simulink model "torqueBalancingSOT_logData"  (Simulink 8.8)
settings: Solver=FixedStepDiscrete  StartTime=0.0  StopTime=CONFIG.SIMULATION_TIME  FixedStep=CONFIG.Ts  RelTol=1e-3  EnableMultiTasking=on
InitFcn:
  | cd(fileparts(which(bdroot)));
  | initTorqueBalancingSOT;
undefined symbols (not defined in the file or in its folder): CONFIG, ConstraintsFeetMatrix, DiscIntNeverNeededParam, gain, reg, ROBOT_DOF, sat, sm, upperBoundFeetConstraints, WBT_robotName
libraries: WBToolboxLibrary x69
(part 2 of 2)

== system torqueBalancingSOT_logData/Visualize and log/Visualize torques ==
  state : Inport
  measuredJointsTorque : Inport  Port=2
  desiredJointsTorque : Inport  Port=3
  Enable : EnablePort
  Add : Sum  Inputs=+-
  DoFs converter : WBToolboxLibrary/Utilities/DoFs converter  yarp2WBIOption=From WBI to YARP  robotName=WBT_robotName  localName=WBT_modelName  wbiFile=WBT_wbiFilename  wbiList=WBT_wbiList
  DoFs converter1 : WBToolboxLibrary/Utilities/DoFs converter  yarp2WBIOption=From WBI to YARP  robotName=WBT_robotName  localName=WBT_modelName  wbiFile=WBT_wbiFilename  wbiList=WBT_wbiList
  DoFs converter2 : WBToolboxLibrary/Utilities/DoFs converter  yarp2WBIOption=From WBI to YARP  robotName=WBT_robotName  localName=WBT_modelName  wbiFile=WBT_wbiFilename  wbiList=WBT_wbiList
  desiredJointTorques : Scope  NumInputPorts=6
  errorJointTorques : Scope  NumInputPorts=6
  measuredJointTorques : Scope  NumInputPorts=6
  wires:
  DoFs converter1/2 -> desiredJointTorques/2  "left_arm"
  DoFs converter2/3 -> errorJointTorques/3  "right_arm"
  DoFs converter2/5 -> errorJointTorques/5  "right_leg"
  DoFs converter2/1 -> errorJointTorques/1  "torso"
  DoFs converter/5 -> measuredJointTorques/5  "right_leg"
  DoFs converter/4 -> measuredJointTorques/4  "left_leg"
  DoFs converter/2 -> measuredJointTorques/2  "left_arm"
  DoFs converter/1 -> measuredJointTorques/1  "torso"
  desiredJointsTorque/1 -> DoFs converter1/1, Add/2
  measuredJointsTorque/1 -> Add/1, DoFs converter/1
  DoFs converter/3 -> measuredJointTorques/3  "right_arm"
  DoFs converter2/4 -> errorJointTorques/4  "left_leg"
  DoFs converter1/1 -> desiredJointTorques/1  "torso"
  DoFs converter1/3 -> desiredJointTorques/3  "right_arm"
  DoFs converter1/4 -> desiredJointTorques/4  "left_leg"
  DoFs converter2/2 -> errorJointTorques/2  "left_arm"
  Add/1 -> DoFs converter2/1
  DoFs converter1/5 -> desiredJointTorques/5  "right_leg"
  state/1 -> measuredJointTorques/6, errorJointTorques/6, desiredJointTorques/6

== system torqueBalancingSOT_logData/synchronizer/GAZEBO_SYNCHRONIZER ==
  Enable : EnablePort
  Simulator Synchronizer : WBToolboxLibrary/Utilities/Simulator Synchronizer  period=CONFIG.Ts  serverPortName='/clock/rpc'  clientPortName='/WBT_synchronizer/rpc:o'

== system torqueBalancingSOT_logData/synchronizer/REAL_TIME_SYNC ==
  Enable : EnablePort
  Real Time Synchronizer : WBToolboxLibrary/Utilities/Real Time Synchronizer  period=CONFIG.Ts

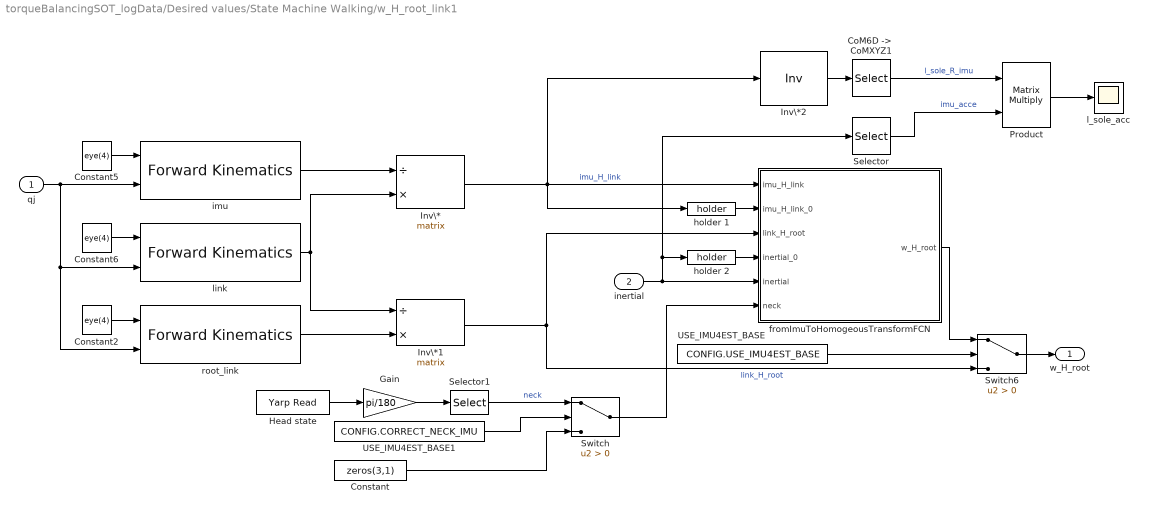
== system torqueBalancingSOT_logData/Desired values/State Machine Walking/w_H_root_link1 ==
  qj : Inport
  inertial : Inport  Port=2
  "CoM6D ->  CoMXYZ1" : Selector  NumberOfDimensions=2  InputPortWidth=7  IndexOptions=Index vector (dialog),Index vector (dialog)  Indices=[1 2 3],[1 2 3]  OutputSizes=1,1
  Constant : Constant  Value=zeros(3,1)
  Constant2 : Constant  Value=eye(4)
  Constant5 : Constant  Value=eye(4)
  Constant6 : Constant  Value=eye(4)
  Gain : Gain  Gain=pi/180
  Head state : WBToolboxLibrary/Utilities/Yarp Read  portName=[WBT_robotName, '/head/state:o']  signalSize=6  blocking=off  timestamp=off  autoconnect=on  errorOnConnection=off
  Inv\* : Product  Inputs=/*  Multiplication=Matrix(*)
  Inv\*1 : Product  Inputs=/*  Multiplication=Matrix(*)
  Inv\*2 : Product  Inputs=/  Multiplication=Matrix(*)
  Product : Product  Multiplication=Matrix(*)
  Selector : Selector  InputPortWidth=12  IndexOptions=Index vector (dialog)  Indices=[4 5 6 ]  OutputSizes=1
  Selector1 : Selector  InputPortWidth=6  IndexOptions=Index vector (dialog)  Indices=[1:3]  OutputSizes=1
  Switch : Switch  Criteria=u2 > Threshold
  Switch6 : Switch  Criteria=u2 > Threshold
  USE_IMU4EST_BASE : Constant  Value=CONFIG.USE_IMU4EST_BASE
  USE_IMU4EST_BASE1 : Constant  Value=CONFIG.CORRECT_NECK_IMU
  fromImuToHomogeousTransformFCN : MATLAB Function  TreatAsAtomicUnit=on
  holder 1 : WBToolboxLibrary/Utilities/holder 
  holder 2 : WBToolboxLibrary/Utilities/holder 
  imu : WBToolboxLibrary/wholeBodyModel/Kinematics/Forward Kinematics  frameName='imu_frame'  robotName=WBT_robotName  localName=WBT_modelName  wbiFile=WBT_wbiFilename  wbiList=WBT_wbiList
  l_sole_acc : Scope
  link : WBToolboxLibrary/wholeBodyModel/Kinematics/Forward Kinematics  frameName=link_name  robotName=WBT_robotName  localName=WBT_modelName  wbiFile=WBT_wbiFilename  wbiList=WBT_wbiList
  root_link : WBToolboxLibrary/wholeBodyModel/Kinematics/Forward Kinematics  frameName=FRAMES.BASE  robotName=WBT_robotName  localName=WBT_modelName  wbiFile=WBT_wbiFilename  wbiList=WBT_wbiList
  w_H_root : Outport
  wires:
  Constant5/1 -> imu/1
  Inv\*/1 -> Inv\*2/1, holder 1/1, fromImuToHomogeousTransformFCN/1(imu_H_link)  "imu_H_link"
  imu/1 -> Inv\*/1
  Constant6/1 -> link/1
  Inv\*1/1 -> Switch6/3, fromImuToHomogeousTransformFCN/3(link_H_root)  "link_H_root"
  link/1 -> Inv\*/2, Inv\*1/1
  inertial/1 -> Selector/1, holder 2/1, fromImuToHomogeousTransformFCN/5(inertial)
  Switch6/1 -> w_H_root/1
  USE_IMU4EST_BASE/1 -> Switch6/2
  fromImuToHomogeousTransformFCN/1(w_H_root) -> Switch6/1
  Constant2/1 -> root_link/1
  qj/1 -> root_link/2, link/2, imu/2
  root_link/1 -> Inv\*1/2
  holder 1/1 -> fromImuToHomogeousTransformFCN/2(imu_H_link_0)
  holder 2/1 -> fromImuToHomogeousTransformFCN/4(inertial_0)
  Inv\*2/1 -> "CoM6D ->  CoMXYZ1"/1
  "CoM6D ->  CoMXYZ1"/1 -> Product/1  "l_sole_R_imu"
  Selector/1 -> Product/2  "imu_acce"
  Product/1 -> l_sole_acc/1
  Head state/1 -> Gain/1
  Selector1/1 -> Switch/1  "neck"
  USE_IMU4EST_BASE1/1 -> Switch/2
  Switch/1 -> fromImuToHomogeousTransformFCN/6(neck)
  Gain/1 -> Selector1/1
  Constant/1 -> Switch/3

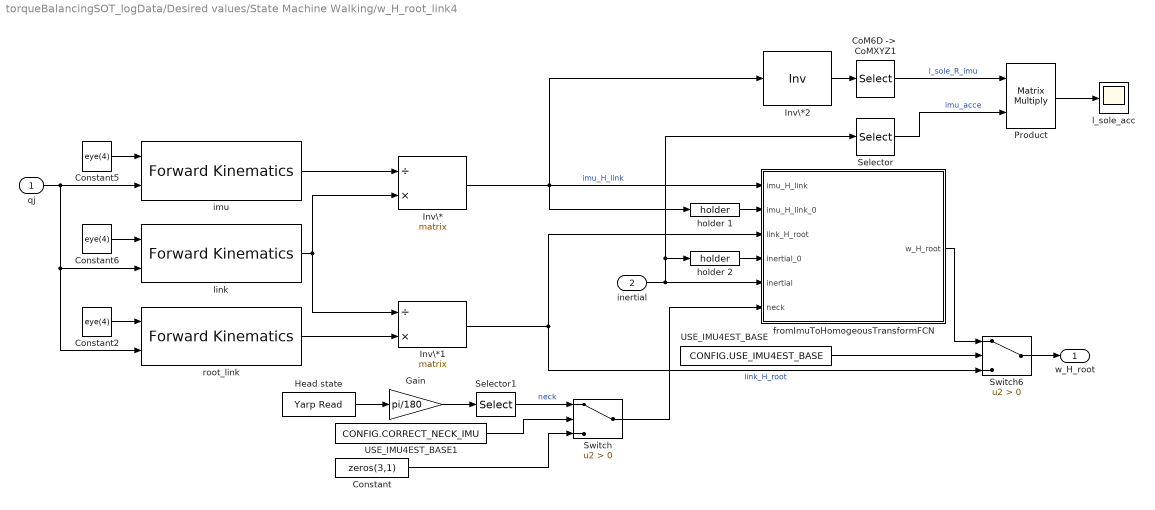
== system torqueBalancingSOT_logData/Desired values/State Machine Walking/w_H_root_link4 ==
  qj : Inport
  inertial : Inport  Port=2
  "CoM6D ->  CoMXYZ1" : Selector  NumberOfDimensions=2  InputPortWidth=7  IndexOptions=Index vector (dialog),Index vector (dialog)  Indices=[1 2 3],[1 2 3]  OutputSizes=1,1
  Constant : Constant  Value=zeros(3,1)
  Constant2 : Constant  Value=eye(4)
  Constant5 : Constant  Value=eye(4)
  Constant6 : Constant  Value=eye(4)
  Gain : Gain  Gain=pi/180
  Head state : WBToolboxLibrary/Utilities/Yarp Read  portName=[WBT_robotName, '/head/state:o']  signalSize=6  blocking=off  timestamp=off  autoconnect=on  errorOnConnection=off
  Inv\* : Product  Inputs=/*  Multiplication=Matrix(*)
  Inv\*1 : Product  Inputs=/*  Multiplication=Matrix(*)
  Inv\*2 : Product  Inputs=/  Multiplication=Matrix(*)
  Product : Product  Multiplication=Matrix(*)
  Selector : Selector  InputPortWidth=12  IndexOptions=Index vector (dialog)  Indices=[4 5 6 ]  OutputSizes=1
  Selector1 : Selector  InputPortWidth=6  IndexOptions=Index vector (dialog)  Indices=[1:3]  OutputSizes=1
  Switch : Switch  Criteria=u2 > Threshold
  Switch6 : Switch  Criteria=u2 > Threshold
  USE_IMU4EST_BASE : Constant  Value=CONFIG.USE_IMU4EST_BASE
  USE_IMU4EST_BASE1 : Constant  Value=CONFIG.CORRECT_NECK_IMU
  fromImuToHomogeousTransformFCN : MATLAB Function  TreatAsAtomicUnit=on
  holder 1 : WBToolboxLibrary/Utilities/holder 
  holder 2 : WBToolboxLibrary/Utilities/holder 
  imu : WBToolboxLibrary/wholeBodyModel/Kinematics/Forward Kinematics  frameName='imu_frame'  robotName=WBT_robotName  localName=WBT_modelName  wbiFile=WBT_wbiFilename  wbiList=WBT_wbiList
  l_sole_acc : Scope
  link : WBToolboxLibrary/wholeBodyModel/Kinematics/Forward Kinematics  frameName=link_name  robotName=WBT_robotName  localName=WBT_modelName  wbiFile=WBT_wbiFilename  wbiList=WBT_wbiList
  root_link : WBToolboxLibrary/wholeBodyModel/Kinematics/Forward Kinematics  frameName=FRAMES.BASE  robotName=WBT_robotName  localName=WBT_modelName  wbiFile=WBT_wbiFilename  wbiList=WBT_wbiList
  w_H_root : Outport
  wires:
  Constant5/1 -> imu/1
  Inv\*/1 -> Inv\*2/1, holder 1/1, fromImuToHomogeousTransformFCN/1(imu_H_link)  "imu_H_link"
  imu/1 -> Inv\*/1
  Constant6/1 -> link/1
  Inv\*1/1 -> Switch6/3, fromImuToHomogeousTransformFCN/3(link_H_root)  "link_H_root"
  link/1 -> Inv\*/2, Inv\*1/1
  inertial/1 -> Selector/1, holder 2/1, fromImuToHomogeousTransformFCN/5(inertial)
  Switch6/1 -> w_H_root/1
  USE_IMU4EST_BASE/1 -> Switch6/2
  fromImuToHomogeousTransformFCN/1(w_H_root) -> Switch6/1
  Constant2/1 -> root_link/1
  qj/1 -> root_link/2, link/2, imu/2
  root_link/1 -> Inv\*1/2
  holder 1/1 -> fromImuToHomogeousTransformFCN/2(imu_H_link_0)
  holder 2/1 -> fromImuToHomogeousTransformFCN/4(inertial_0)
  Inv\*2/1 -> "CoM6D ->  CoMXYZ1"/1
  "CoM6D ->  CoMXYZ1"/1 -> Product/1  "l_sole_R_imu"
  Selector/1 -> Product/2  "imu_acce"
  Product/1 -> l_sole_acc/1
  Head state/1 -> Gain/1
  Selector1/1 -> Switch/1  "neck"
  USE_IMU4EST_BASE1/1 -> Switch/2
  Switch/1 -> fromImuToHomogeousTransformFCN/6(neck)
  Gain/1 -> Selector1/1
  Constant/1 -> Switch/3

== system torqueBalancingSOT_logData/Desired values/State Machine Walking/xCom ==
  qj : Inport
  w_H_b : Inport  Port=2
  "CoM6D ->  CoMXYZ2" : Selector  NumberOfDimensions=2  InputPortWidth=7  IndexOptions=Index vector (dialog),Index vector (dialog)  Indices=[1 2 3],[4]  OutputSizes=1,1
  com : WBToolboxLibrary/wholeBodyModel/Kinematics/Forward Kinematics  frameName='com'  robotName=WBT_robotName  localName=WBT_modelName  wbiFile=WBT_wbiFilename  wbiList=WBT_wbiList
  xCom : Outport
  wires:
  qj/1 -> com/2
  "CoM6D ->  CoMXYZ2"/1 -> xCom/1
  com/1 -> "CoM6D ->  CoMXYZ2"/1
  w_H_b/1 -> com/1

== system torqueBalancingSOT_logData/Desired values/State Machine Walking/xCom1 ==
  qj : Inport
  w_H_b : Inport  Port=2
  "CoM6D ->  CoMXYZ2" : Selector  NumberOfDimensions=2  InputPortWidth=7  IndexOptions=Index vector (dialog),Index vector (dialog)  Indices=[1 2 3],[4]  OutputSizes=1,1
  com : WBToolboxLibrary/wholeBodyModel/Kinematics/Forward Kinematics  frameName='com'  robotName=WBT_robotName  localName=WBT_modelName  wbiFile=WBT_wbiFilename  wbiList=WBT_wbiList
  xCom : Outport
  wires:
  w_H_b/1 -> com/1
  com/1 -> "CoM6D ->  CoMXYZ2"/1
  "CoM6D ->  CoMXYZ2"/1 -> xCom/1
  qj/1 -> com/2

== system torqueBalancingSOT_logData/Integration Based Inverse Kinematics/referenceAccelerations/Jacobians ==
  w_H_b : Inport
  JointAngles : Inport  Port=2
  baseVelocity : Inport  Port=3
  jointVelocity : Inport  Port=4
  DotJ Nu : WBToolboxLibrary/wholeBodyModel/Jacobians/DotJ Nu  frameName='com'  robotName=WBT_robotName  localName=WBT_modelName  wbiFile=WBT_wbiFilename  wbiList=WBT_wbiList
  DotJ Nu1 : WBToolboxLibrary/wholeBodyModel/Jacobians/DotJ Nu  frameName='root_link'  robotName=WBT_robotName  localName=WBT_modelName  wbiFile=WBT_wbiFilename  wbiList=WBT_wbiList
  DotJ Nu2 : WBToolboxLibrary/wholeBodyModel/Jacobians/DotJ Nu  frameName='l_sole'  robotName=WBT_robotName  localName=WBT_modelName  wbiFile=WBT_wbiFilename  wbiList=WBT_wbiList
  DotJ Nu3 : WBToolboxLibrary/wholeBodyModel/Jacobians/DotJ Nu  frameName='r_sole'  robotName=WBT_robotName  localName=WBT_modelName  wbiFile=WBT_wbiFilename  wbiList=WBT_wbiList
  Jacobian1 : WBToolboxLibrary/wholeBodyModel/Jacobians/Jacobian  frameName='com'  robotName=WBT_robotName  localName=WBT_modelName  wbiFile=WBT_wbiFilename  wbiList=WBT_wbiList
  Jacobian2 : WBToolboxLibrary/wholeBodyModel/Jacobians/Jacobian  frameName='root_link'  robotName=WBT_robotName  localName=WBT_modelName  wbiFile=WBT_wbiFilename  wbiList=WBT_wbiList
  Jacobian3 : WBToolboxLibrary/wholeBodyModel/Jacobians/Jacobian  frameName='l_sole'  robotName=WBT_robotName  localName=WBT_modelName  wbiFile=WBT_wbiFilename  wbiList=WBT_wbiList
  Jacobian4 : WBToolboxLibrary/wholeBodyModel/Jacobians/Jacobian  frameName='r_sole'  robotName=WBT_robotName  localName=WBT_modelName  wbiFile=WBT_wbiFilename  wbiList=WBT_wbiList
  Matrix Concatenate1 : Concatenate  NumInputs=4  Mode=Multidimensional array
  Matrix Concatenate2 : Concatenate  NumInputs=4  Mode=Multidimensional array
  Selector2 : Selector  NumberOfDimensions=2  InputPortWidth=6+ROBOT_DOF  IndexOptions=Index vector (dialog),Index vector (dialog)  Indices=[4:6],[1:6+ROBOT_DOF]  OutputSizes=1,1
  Selector3 : Selector  NumberOfDimensions=2  InputPortWidth=6+ROBOT_DOF  IndexOptions=Index vector (dialog),Index vector (dialog)  Indices=[1:3],[1:6+ROBOT_DOF]  OutputSizes=1,1
  Selector4 : Selector  InputPortWidth=6  IndexOptions=Index vector (dialog)  Indices=[1:3]  OutputSizes=1
  Selector5 : Selector  InputPortWidth=6  IndexOptions=Index vector (dialog)  Indices=[4:6]  OutputSizes=1
  Jtask : Outport
  dJNu_task : Outport  Port=2
  wires:
  Jacobian1/1 -> Selector3/1
  jointVelocity/1 -> DotJ Nu1/4, DotJ Nu2/4, DotJ Nu3/4, DotJ Nu/4
  Jacobian2/1 -> Selector2/1
  Selector5/1 -> Matrix Concatenate2/2
  DotJ Nu2/1 -> Matrix Concatenate2/3
  Matrix Concatenate2/1 -> dJNu_task/1
  DotJ Nu3/1 -> Matrix Concatenate2/4
  Jacobian4/1 -> Matrix Concatenate1/4
  DotJ Nu/1 -> Selector4/1
  Selector4/1 -> Matrix Concatenate2/1
  Jacobian3/1 -> Matrix Concatenate1/3
  w_H_b/1 -> Jacobian1/1, Jacobian2/1, Jacobian3/1, Jacobian4/1, DotJ Nu/1, DotJ Nu1/1, DotJ Nu2/1, DotJ Nu3/1
  JointAngles/1 -> Jacobian2/2, Jacobian3/2, Jacobian4/2, DotJ Nu/2, DotJ Nu1/2, DotJ Nu2/2, DotJ Nu3/2, Jacobian1/2
  DotJ Nu1/1 -> Selector5/1
  baseVelocity/1 -> DotJ Nu/3, DotJ Nu1/3, DotJ Nu2/3, DotJ Nu3/3
  Selector3/1 -> Matrix Concatenate1/1
  Matrix Concatenate1/1 -> Jtask/1
  Selector2/1 -> Matrix Concatenate1/2

== system torqueBalancingSOT_logData/Integration Based Inverse Kinematics/referenceAccelerations/Kinematics ==
  w_H_b : Inport
  JointAngles : Inport  Port=2
  Forward KinematicsCoM : WBToolboxLibrary/wholeBodyModel/Kinematics/Forward Kinematics  frameName='com'  robotName=WBT_robotName  localName=WBT_modelName  wbiFile=WBT_wbiFilename  wbiList=WBT_wbiList
  Forward KinematicsCoM1 : WBToolboxLibrary/wholeBodyModel/Kinematics/Forward Kinematics  frameName='root_link'  robotName=WBT_robotName  localName=WBT_modelName  wbiFile=WBT_wbiFilename  wbiList=WBT_wbiList
  Forward Kinematics_lFoot : WBToolboxLibrary/wholeBodyModel/Kinematics/Forward Kinematics  frameName='l_sole'  robotName=WBT_robotName  localName=WBT_modelName  wbiFile=WBT_wbiFilename  wbiList=WBT_wbiList
  Forward Kinematics_rFoot : WBToolboxLibrary/wholeBodyModel/Kinematics/Forward Kinematics  frameName='r_sole'  robotName=WBT_robotName  localName=WBT_modelName  wbiFile=WBT_wbiFilename  wbiList=WBT_wbiList
  Selector : Selector  NumberOfDimensions=2  InputPortWidth=6+ROBOT_DOF  IndexOptions=Index vector (dialog),Index vector (dialog)  Indices=[1:3],[4]  OutputSizes=1,1
  Selector1 : Selector  NumberOfDimensions=2  InputPortWidth=9  IndexOptions=Index vector (dialog),Index vector (dialog)  Indices=[1:3],[1:3]  OutputSizes=1,1
  CoMPos : Outport
  w_R_root : Outport  Port=2
  w_H_lsole : Outport  Port=3
  w_H_rsole : Outport  Port=4
  wires:
  JointAngles/1 -> Forward Kinematics_rFoot/2, Forward Kinematics_lFoot/2, Forward KinematicsCoM1/2, Forward KinematicsCoM/2
  Selector1/1 -> w_R_root/1
  Forward Kinematics_lFoot/1 -> w_H_lsole/1
  Forward Kinematics_rFoot/1 -> w_H_rsole/1
  Forward KinematicsCoM/1 -> Selector/1
  Selector/1 -> CoMPos/1
  Forward KinematicsCoM1/1 -> Selector1/1
  w_H_b/1 -> Forward Kinematics_rFoot/1, Forward Kinematics_lFoot/1, Forward KinematicsCoM1/1, Forward KinematicsCoM/1

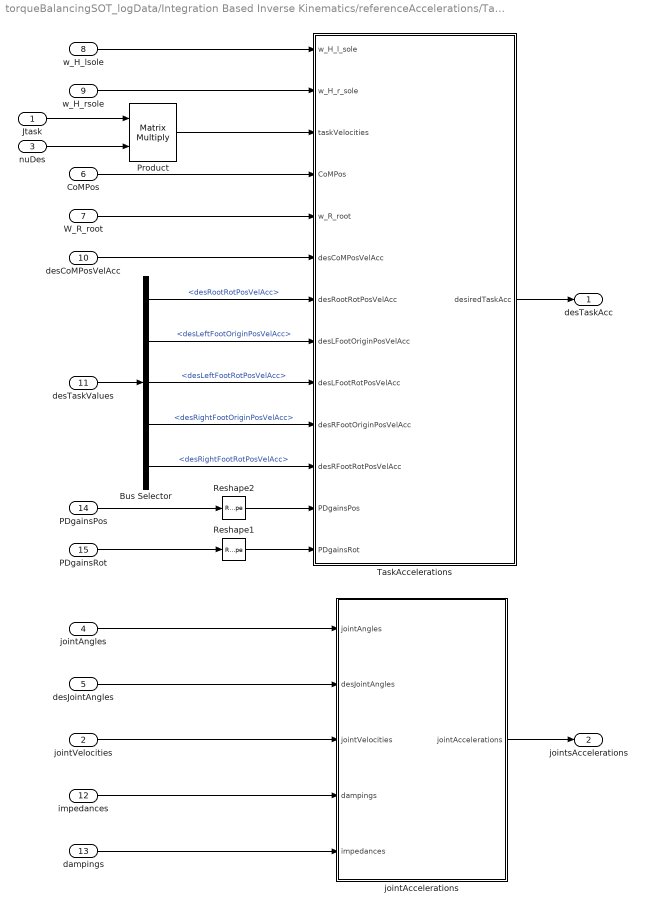
== system torqueBalancingSOT_logData/Integration Based Inverse Kinematics/referenceAccelerations/Task and Joint Accelerations ==
  Jtask : Inport
  jointVelocities : Inport  Port=2
  nuDes : Inport  Port=3
  jointAngles : Inport  Port=4
  desJointAngles : Inport  Port=5
  CoMPos : Inport  Port=6
  W_R_root : Inport  Port=7
  w_H_lsole : Inport  Port=8
  w_H_rsole : Inport  Port=9
  desCoMPosVelAcc : Inport  Port=10
  desTaskValues : Inport  Port=11
  impedances : Inport  Port=12
  dampings : Inport  Port=13
  PDgainsPos : Inport  Port=14
  PDgainsRot : Inport  Port=15
  Bus Selector : BusSelector  OutputSignals=desRootRotPosVelAcc,desLeftFootOriginPosVelAcc,desLeftFootRotPosVelAcc,desRightFootOriginPosVelAcc,desRightFootRotPosVelAcc
  Product : Product  Multiplication=Matrix(*)
  Reshape1 : Reshape  OutputDimensionality=Customize  OutputDimensions=[3,2]
  Reshape2 : Reshape  OutputDimensionality=Customize  OutputDimensions=[1,18]
  TaskAccelerations : MATLAB Function  TreatAsAtomicUnit=on
  jointAccelerations : MATLAB Function  TreatAsAtomicUnit=on
  desTaskAcc : Outport
  jointsAccelerations : Outport  Port=2
  wires:
  nuDes/1 -> Product/2
  desCoMPosVelAcc/1 -> TaskAccelerations/6(desCoMPosVelAcc)
  Bus Selector/5 -> TaskAccelerations/11(desRFootRotPosVelAcc)  "<desRightFootRotPosVelAcc>"
  desTaskValues/1 -> Bus Selector/1
  Bus Selector/3 -> TaskAccelerations/9(desLFootRotPosVelAcc)  "<desLeftFootRotPosVelAcc>"
  jointAngles/1 -> jointAccelerations/1(jointAngles)
  Bus Selector/2 -> TaskAccelerations/8(desLFootOriginPosVelAcc)  "<desLeftFootOriginPosVelAcc>"
  Bus Selector/1 -> TaskAccelerations/7(desRootRotPosVelAcc)  "<desRootRotPosVelAcc>"
  W_R_root/1 -> TaskAccelerations/5(w_R_root)
  CoMPos/1 -> TaskAccelerations/4(CoMPos)
  TaskAccelerations/1(desiredTaskAcc) -> desTaskAcc/1
  Jtask/1 -> Product/1
  jointVelocities/1 -> jointAccelerations/3(jointVelocities)
  jointAccelerations/1(jointAccelerations) -> jointsAccelerations/1
  Bus Selector/4 -> TaskAccelerations/10(desRFootOriginPosVelAcc)  "<desRightFootOriginPosVelAcc>"
  desJointAngles/1 -> jointAccelerations/2(desJointAngles)
  Product/1 -> TaskAccelerations/3(taskVelocities)
  w_H_rsole/1 -> TaskAccelerations/2(w_H_r_sole)
  w_H_lsole/1 -> TaskAccelerations/1(w_H_l_sole)
  PDgainsPos/1 -> Reshape2/1
  PDgainsRot/1 -> Reshape1/1
  impedances/1 -> jointAccelerations/4(dampings)
  dampings/1 -> jointAccelerations/5(impedances)
  Reshape2/1 -> TaskAccelerations/12(PDgainsPos)
  Reshape1/1 -> TaskAccelerations/13(PDgainsRot)

== matlab function Integration Based Inverse Kinematics/referenceAccelerations/Task and Joint Accelerations/jointAccelerations ==
  data: jointAngles input double; desJointAngles input double; jointVelocities input double; jointAccelerations output double; dampings input double; impedances input double
function jointAccelerations = jointDynamicsFCN(jointAngles, desJointAngles, jointVelocities, dampings, impedances)
                            
jointAccelerations = jointDynamics(jointAngles, desJointAngles, jointVelocities, impedances, dampings);

== matlab function Desired values/State Machine Walking/stateMachineWalkingFCN ==
  data: t input double; qDes output double; qj input double; qj0 input double; CoM_0 input double; l_sole_CoM input double; r_sole_CoM input double; l_sole_H_b input double; r_sole_H_b input double; wrench_leftFoot input double; wrench_rightFoot input double; CoMDes output double; desRootRotPosVelAcc output double; desLeftFootOriginPos output double; desLeftFootRotPosVelAcc output double; desRightFootOriginPos output double; desRightFootRotPosVelAcc output double; impedances output double; dampings output double; PDgainsPos output double; PDgainsRot output double; jointsSmoothingTime output double; w_H_b output double; feetConstraints output double; currentState output double; sm parameter double; gain parameter double
function [qDes, CoMDes, desRootRotPosVelAcc, ...
          desLeftFootOriginPos, desLeftFootRotPosVelAcc, desRightFootOriginPos, desRightFootRotPosVelAcc,  ...
          impedances, dampings, PDgainsPos, PDgainsRot, jointsSmoothingTime, w_H_b, feetConstraints, currentState] ...
          = stateMachineWalkingFCN(t, qj, qj0, CoM_0, ...
                                   l_sole_CoM, r_sole_CoM, l_sole_H_b, r_sole_H_b, ...
                                   wrench_leftFoot, wrench_rightFoot, sm, gain)

[w_H_b, CoMDes, qDes,feetConstraints, impedances, dampings, PDgainsPos, PDgainsRot, currentState, jointsSmoothingTime,...
 desRootRotPosVelAcc, desLeftFootRotPosVelAcc, desLeftFootOriginPos, desRightFootRotPosVelAcc, desRightFootOriginPos] ...
= stateMachineWalking(t, qj, qj0, CoM_0, ...
                      l_sole_CoM, r_sole_CoM, l_sole_H_b, r_sole_H_b, ...
                      wrench_leftFoot, wrench_rightFoot, sm, gain);

== matlab function Dynamics, Kinematics, Jacobians/Jacobians/baseVelocityFCN ==
  data: JcLeftFoot input double; vb output double; JcRightFoot input double; feetConstraints input double; dqj input double; reg parameter double
function vb = baseVelocityFCN(JcLeftFoot, JcRightFoot, feetConstraints, dqj, reg)

vb = baseVelocity(JcLeftFoot, JcRightFoot, feetConstraints, dqj, reg);

== matlab function Visualize and log/Visualize tasks/MATLAB Function ==
  data: errorVector input double; error output double
function error = norm(errorVector)

error = norm(errorVector);

== matlab function Integration Based Inverse Kinematics/referenceAccelerations/Task and Joint Accelerations/TaskAccelerations ==
  data: w_H_l_sole input double; w_H_r_sole input double; taskVelocities input double; CoMPos input double; w_R_root input double; desCoMPosVelAcc input double; desiredTaskAcc output double; desRootRotPosVelAcc input double; desLFootOriginPosVelAcc input double; desLFootRotPosVelAcc input double; desRFootOriginPosVelAcc input double; desRFootRotPosVelAcc input double; PDgainsPos input double; PDgainsRot input double
function desiredTaskAcc   = desiredTaskAccelerationFCN...
         (w_H_l_sole,w_H_r_sole, taskVelocities, CoMPos, w_R_root,...
         desCoMPosVelAcc,         desRootRotPosVelAcc, ...
         desLFootOriginPosVelAcc, desLFootRotPosVelAcc, ...
         desRFootOriginPosVelAcc, desRFootRotPosVelAcc, ...
         PDgainsPos, PDgainsRot)     
     
     [desiredTaskAcc,~,~,~,~,~,~,~] = desiredTaskAcceleration(w_H_l_sole, w_H_r_sole, taskVelocities, CoMPos, w_R_root,...
                                      desCoMPosVelAcc, desRootRotPosVelAcc,...
                                      desLFootOriginPosVelAcc, desLFootRotPosVelAcc, ...
                                      desRFootOriginPosVelAcc, desRFootRotPosVelAcc, ...
                                      PDgainsPos, PDgainsRot);
                                            
end

== matlab function Task Acceleration/desiredTaskAcceleration ==
  data: w_H_l_sole input double; w_H_r_sole input double; taskVelocities input double; CoMPos input double; fixedLink_R_root input double; desCoMPosVelAcc input double; desRootRotPosVelAcc input double; desLeftFootOriginPosVelAcc input double; desLeftFootRotPosVelAcc input double; desRightFootOriginPosVelAcc input double; desRightFootRotPosVelAcc input double; PDgainsPos input double; PDgainsRot input double; desiredTaskAcc output double; rootRotError output double; leftFootOriginError output double; leftFootRotError output double; rightFootOriginError output double; rightFootRotError output double
function [desiredTaskAcc, rootRotError, leftFootOriginError, leftFootRotError, rightFootOriginError, rightFootRotError] = ...
    desiredTaskAccelerationFCN(w_H_l_sole, w_H_r_sole, taskVelocities, CoMPos, fixedLink_R_root,...
                               desCoMPosVelAcc, desRootRotPosVelAcc,...
                               desLeftFootOriginPosVelAcc,  desLeftFootRotPosVelAcc, ...
                               desRightFootOriginPosVelAcc, desRightFootRotPosVelAcc, ...
                               PDgainsPos, PDgainsRot)
                           
 [desiredTaskAcc, ~, rootRotError, leftFootOriginError, leftFootRotError, rightFootOriginError, rightFootRotError, ~] = ...
              desiredTaskAcceleration(w_H_l_sole, w_H_r_sole, taskVelocities, CoMPos, fixedLink_R_root,...
                                      desCoMPosVelAcc, desRootRotPosVelAcc,...
                                      desLeftFootOriginPosVelAcc,  desLeftFootRotPosVelAcc, ...
                                      desRightFootOriginPosVelAcc, desRightFootRotPosVelAcc, ...
                                      PDgainsPos, PDgainsRot);

== matlab function Controller and QP/balancingController ==
  data: feetConstraints input double; impedances input double; dampings input double; qj input double; hessianMatrix output double; M input double; h input double; dJcNu input double; w_H_l_sole input double; w_H_r_sole input double; Jc input double; nu input double; desiredJointAngles input double; desiredTaskAcc input double; biasVector output double; constraintMatrixLeftFoot output double; constraintMatrixRightFoot output double; constraintMatrixEq output double; upperBoundEqConstraints output double; ROBOT_DOF_FOR_SIMULINK input double; ConstraintsFeetMatrix input double; gain parameter double; CONFIG parameter double
function [hessianMatrix, biasVector, ...
          constraintMatrixLeftFoot, constraintMatrixRightFoot, ...
          constraintMatrixEq, upperBoundEqConstraints] = ...
          balancingControllerSOT_FCN(feetConstraints, impedances, dampings, qj, ...
                                     M, h, dJcNu, w_H_l_sole, w_H_r_sole, Jc, nu, ...
                                     desiredJointAngles, desiredTaskAcc, ...
                                     ROBOT_DOF_FOR_SIMULINK, ConstraintsFeetMatrix, ...
                                     gain, CONFIG)

[hessianMatrix,biasVector,constraintMatrixLeftFoot,constraintMatrixRightFoot,constraintMatrixEq, upperBoundEqConstraints] = ...
                                        balancingControllerSOT(feetConstraints, impedances, dampings, qj, ...
                                                               M, h, dJcNu, w_H_l_sole, w_H_r_sole, Jc, nu, ...
                                                               desiredJointAngles, desiredTaskAcc, ...
                                                               ROBOT_DOF_FOR_SIMULINK, ConstraintsFeetMatrix, ...
                                                               gain, CONFIG);

== matlab function Integration Based Inverse Kinematics/referenceAccelerations/trajectoryGeneratorCoM2 ==
  data: Jtask input double; dJnuDes input double; taskAccelerations input double; jointDynamics input double; dnuDes output double; constraints input double; ROBOT_DOF parameter double; reg parameter double
function dnuDes   = referenceAccelerationFCN(Jtask, dJnuDes, taskAccelerations, jointDynamics, ... 
                                                      constraints, ROBOT_DOF, reg)
                                          
dnuDes   = referenceAcceleration(Jtask, dJnuDes, taskAccelerations, jointDynamics, ... 
                                 constraints, ROBOT_DOF, reg);

== matlab function Visualize and log/Visualize tasks/MATLAB Function1 ==
  data: errorVector input double; error output double
function error = norm(errorVector)

error = norm(errorVector);

== matlab function Visualize and log/Visualize tasks/MATLAB Function2 ==
  data: errorVector input double; error output double
function error = norm(errorVector)

error = norm(errorVector);

== matlab function Integration Based Inverse Kinematics/inverse kinematics integration/baseDerivative ==
  data: basePose input double; nuDes_base input double; baseDer output double
function baseDer   = baseDerivative(basePose, nuDes_base)

% Time derivative of the floating base pose. The base orientation is in quaternions
baseDer            = baseDerivative(nuDes_base,basePose);

end

== matlab function Integration Based Inverse Kinematics/inverse kinematics integration/rewrite the base pose as pos+quat ==
  data: qInitQuat input double; qInit output double
function qInit = transfMatrixToQuaternions(qInitQuat)

% Converts the floating base in the initial state vector [16+ndof;1] to 
% position + quaternion representation 
qInit = transfMatrixToQuaternions(qInitQuat);

end

== matlab function Integration Based Inverse Kinematics/inverse kinematics integration/rewrite the base pose as transformation matrix ==
  data: qDesQuat input double; qDes output double
function qDes = fromQuaternionsToTransfMatr(qDesQuat)

% Converts the floating base pose from a quaternion representation to a 
% tranformation matrix
qDes = fromQuaternionsToTransfMatr(qDesQuat);

end

== matlab function Desired values/State Machine Walking/w_H_root_link1/fromImuToHomogeousTransformFCN ==
  data: imu_H_link input double; imu_H_link_0 input double; link_H_root input double; inertial_0 input double; inertial input double; neck input double; w_H_root output double; CONFIG parameter double
function w_H_root = fromBaseToWorldWithImuFCN(imu_H_link,imu_H_link_0,link_H_root,inertial_0,inertial,neck,CONFIG)
%#codegen
w_H_root = fromBaseToWorldWithImu(imu_H_link,imu_H_link_0,link_H_root,inertial_0,inertial,neck,CONFIG);

== matlab function Desired values/State Machine Walking/w_H_root_link4/fromImuToHomogeousTransformFCN ==
  data: imu_H_link input double; imu_H_link_0 input double; link_H_root input double; inertial_0 input double; inertial input double; neck input double; w_H_root output double; CONFIG parameter double
function w_H_root = fromBaseToWorldWithImuFCN(imu_H_link,imu_H_link_0,link_H_root,inertial_0,inertial,neck,CONFIG)
%#codegen
w_H_root = fromBaseToWorldWithImu(imu_H_link,imu_H_link_0,link_H_root,inertial_0,inertial,neck,CONFIG);
